simulink model "pseudoinverse"  (R2020b)
settings: Solver=VariableStepAuto  StartTime=0.0  StopTime=4  RelTol=1e-3
undefined symbols (not defined in the file or in its folder): DiscIntNeverNeededParam
settings Model: Creator=martin  LastModifiedBy=martin

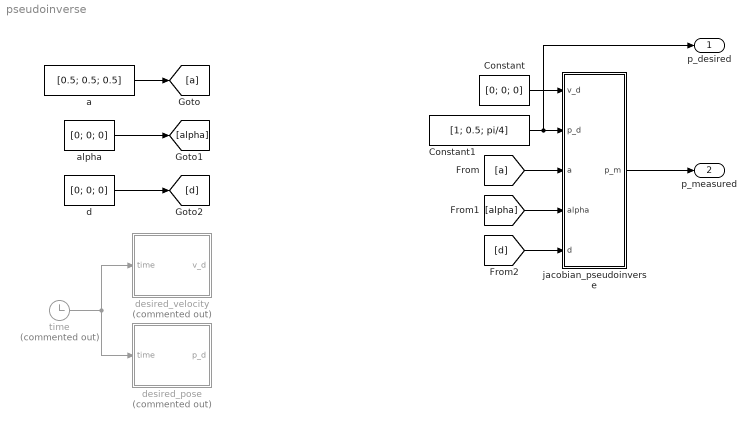
== system pseudoinverse ==
  Constant : Constant  Value=[0; 0; 0]
  Constant1 : Constant  Value=[1; 0.5; pi/4]
  a : Constant  Value=[0.5; 0.5; 0.5]
  alpha : Constant  Value=[0; 0; 0]
  d : Constant  Value=[0; 0; 0]
  desired_pose : Subsystem  Commented=on
  desired_velocity : Subsystem  Commented=on
  jacobian_pseudoinverse : Subsystem
  time : Clock  Commented=on
  p_desired : Outport
  p_measured : Outport  Port=2
  wires:
  time/1 -> desired_pose/1(time), desired_velocity/1(time)
  a/1 -> [a]
  alpha/1 -> [alpha]
  d/1 -> [d]
  [a] -> jacobian_pseudoinverse/3(a)
  [alpha] -> jacobian_pseudoinverse/4(alpha)
  [d] -> jacobian_pseudoinverse/5(d)
  jacobian_pseudoinverse/1(p_m) -> p_measured/1
  Constant/1 -> jacobian_pseudoinverse/1(v_d)
  Constant1/1 -> p_desired/1, jacobian_pseudoinverse/2(p_d)

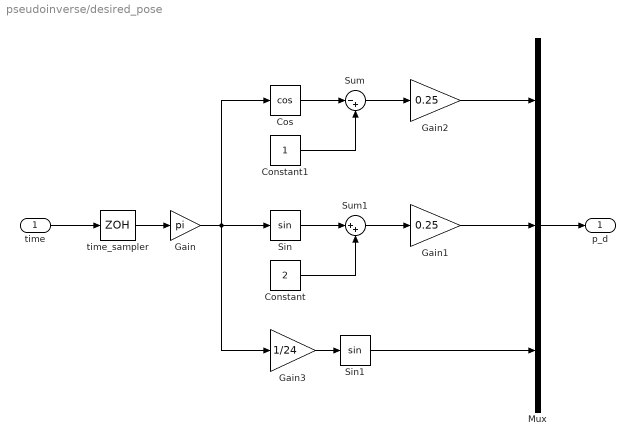
== system pseudoinverse/desired_pose ==
  time : Inport
  Constant : Constant  Value=2
  Constant1 : Constant
  Cos : Trigonometry  Operator=cos
  Gain : Gain  Gain=pi
  Gain1 : Gain  Gain=0.25
  Gain2 : Gain  Gain=0.25
  Gain3 : Gain  Gain=1/24
  Mux : Mux  Inputs=3
  Sin : Trigonometry
  Sin1 : Trigonometry
  Sum : Sum  Inputs=|-+
  Sum1 : Sum  Inputs=|++
  time_sampler : ZeroOrderHold  SampleTime=1e-3
  p_d : Outport
  wires:
  Mux/1 -> p_d/1
  Cos/1 -> Sum/1
  Sum/1 -> Gain2/1
  Constant1/1 -> Sum/2
  Gain/1 -> Gain3/1, Sin/1, Cos/1
  Sin1/1 -> Mux/3
  Gain2/1 -> Mux/1
  Gain3/1 -> Sin1/1
  Gain1/1 -> Mux/2
  Sin/1 -> Sum1/1
  Constant/1 -> Sum1/2
  Sum1/1 -> Gain1/1
  time_sampler/1 -> Gain/1
  time/1 -> time_sampler/1

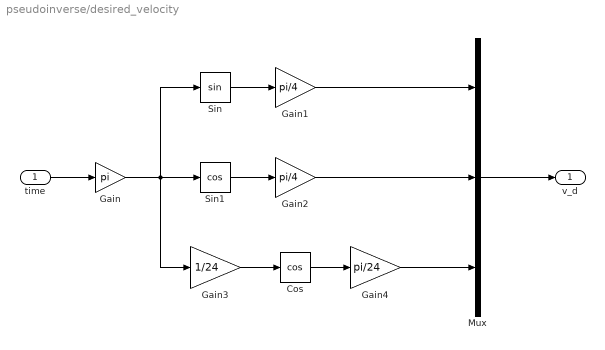
== system pseudoinverse/desired_velocity ==
  time : Inport
  Cos : Trigonometry  Operator=cos
  Gain : Gain  Gain=pi
  Gain1 : Gain  Gain=pi/4
  Gain2 : Gain  Gain=pi/4
  Gain3 : Gain  Gain=1/24
  Gain4 : Gain  Gain=pi/24
  Mux : Mux  Inputs=3
  Sin : Trigonometry
  Sin1 : Trigonometry  Operator=cos
  v_d : Outport
  wires:
  time/1 -> Gain/1
  Gain/1 -> Gain3/1, Sin1/1, Sin/1
  Sin/1 -> Gain1/1
  Sin1/1 -> Gain2/1
  Gain3/1 -> Cos/1
  Cos/1 -> Gain4/1
  Gain1/1 -> Mux/1
  Gain2/1 -> Mux/2
  Mux/1 -> v_d/1
  Gain4/1 -> Mux/3

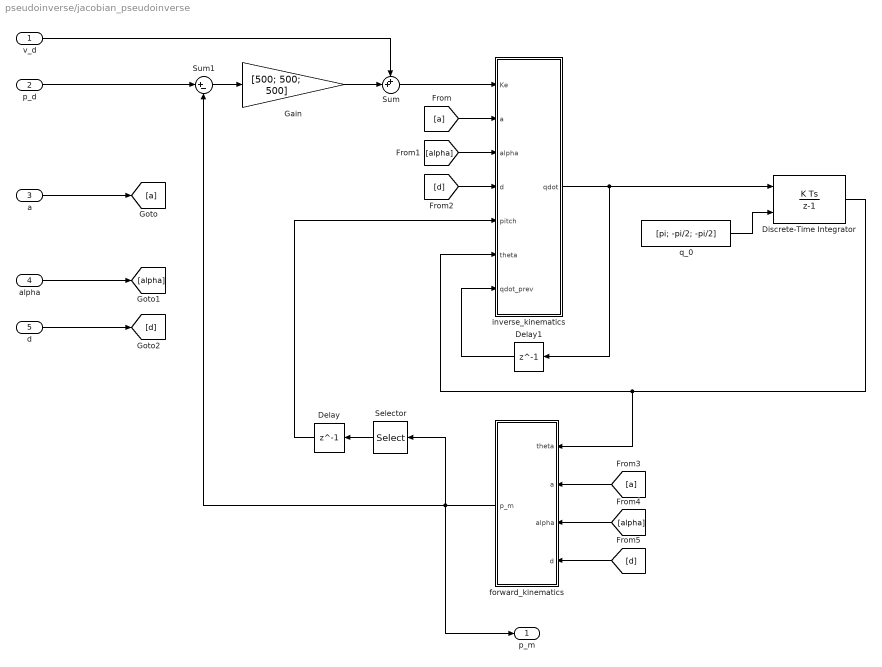
== system pseudoinverse/jacobian_pseudoinverse ==
  v_d : Inport
  p_d : Inport  Port=2
  a : Inport  Port=3
  alpha : Inport  Port=4
  d : Inport  Port=5
  Delay : Delay  DelayLength=1
  Delay1 : Delay  DelayLength=1  SampleTime=1e-3
  Discrete-Time Integrator : DiscreteIntegrator  InitialConditionSource=external  SampleTime=1e-3  ICPrevOutput=DiscIntNeverNeededParam  ICPrevScaledInput=DiscIntNeverNeededParam
  Gain : Gain  Gain=[500; 500; 500]
  Selector : Selector  InputPortWidth=3  IndexOptions=Index vector (dialog)  Indices=[3]  OutputSizes=1
  Sum : Sum  Inputs=++|
  Sum1 : Sum  Inputs=|+-
  forward_kinematics : MATLAB Function  TreatAsAtomicUnit=on
  inverse_kinematics : MATLAB Function  TreatAsAtomicUnit=on
  q_0 : Constant  Value=[pi; -pi/2; -pi/2]
  p_m : Outport
  wires:
  [alpha] -> inverse_kinematics/3(alpha)
  Discrete-Time Integrator/1 -> forward_kinematics/1(theta), inverse_kinematics/6(theta)
  [alpha] -> forward_kinematics/3(alpha)
  inverse_kinematics/1(qdot) -> Discrete-Time Integrator/1, Delay1/1
  [d] -> inverse_kinematics/4(d)
  [a] -> forward_kinematics/2(a)
  [a] -> inverse_kinematics/2(a)
  [d] -> forward_kinematics/4(d)
  q_0/1 -> Discrete-Time Integrator/2
  a/1 -> [a]
  alpha/1 -> [alpha]
  d/1 -> [d]
  p_d/1 -> Sum1/1
  forward_kinematics/1(p_m) -> Sum1/2, p_m/1, Selector/1
  Sum1/1 -> Gain/1
  Selector/1 -> Delay/1
  Delay/1 -> inverse_kinematics/5(pitch)
  Delay1/1 -> inverse_kinematics/7(qdot_prev)
  Gain/1 -> Sum/2
  Sum/1 -> inverse_kinematics/1(Ke)
  v_d/1 -> Sum/1

== matlab function pseudoinverse/jacobian_pseudoinverse/forward_kinematics ==
  data: theta input; a input; alpha input; d input; p_m output
function p_m = fcn(theta, a, alpha, d)
joint_type = ['r'; 'r'; 'r'];
s = forward_kinematics(joint_type, theta, a, alpha, d);
x = s.end_effector_pose();
p_m = [x(1:2,:); x(6,:)];

== matlab function pseudoinverse/jacobian_pseudoinverse/inverse_kinematics ==
  data: Ke input; a input; alpha input; d input; pitch input; qdot output; theta input; qdot_prev input size=[3,1]
function qdot = fcn(Ke, a, alpha, d, pitch, theta, qdot_prev)
joint_type = ['r'; 'r'; 'r'];
s = forward_kinematics(joint_type, theta, a, alpha, d);
J = s.analytical_jacobian(0, pitch);
J_min = [J(1:2,:); J(6,:)];
J_inv = (transpose(J_min)/(J_min*transpose(J_min)));
qdot = J_inv*Ke + (eye(3,3) - J_inv*J_min)*qdot_prev;
